simulink library "Lib_Dyn_StateSpace_TMATS"  (R2017a)
settings: Solver=ode45  StartTime=0.0  StopTime=10.0  RelTol=1e-3  EnableMultiTasking=on
Description:
  | Thomas Modules
settings Model: Creator=jwchapm2  LastModifiedBy=glthoma1
settings DataIOCC: LimitDataPoints=on  SaveFormat=Array
settings OptimizationCC: ExpressionDepthLimit=2147483647  LifeSpan=inf
settings DebuggingCC: UnderspecifiedInitializationDetection=Classic  MergeDetectMultiDrivingBlocksExec=none  SolverPrmCheckMsg=warning  StateNameClashWarn=warning  SFUnexpectedBacktrackingDiag=warning  SFNoUnconditionalDefaultTransitionDiag=warning  SFExecutionAtInitializationDiag=none
settings HardwareCC: ProdBitPerPointer=32  ProdBitPerSizeT=32  ProdBitPerPtrDiffT=32  ProdLargestAtomicFloat=None  ProdIntDivRoundTo=Undefined  ProdEndianess=Unspecified  ProdWordSize=32  ProdHWDeviceType=32-bit Generic
settings ModelReferenceCC: PropagateSignalLabelsOutOfModel=off
settings GRTTargetCC: TargetLangStandard=C89/C90 (ANSI)  GeneratePreprocessorConditionals=Disable all
settings ConfigComp: CovMetricSettings=dw  CovHtmlReporting=on  CovSaveCumulativeToWorkspaceVar=on  CovSaveSingleToWorkspaceVar=on  CovExternalEMLEnable=off

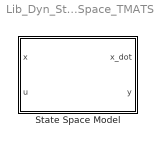
== system Lib_Dyn_StateSpace_TMATS ==
  State Space Model : Subsystem  mask(State Space Model){A_M=-1, B_M=1, C_M=1, D_M=0}
      mask prompts: A_M "A_M - "A" Matrix"; B_M "B_M - "B" Matrix"; C_M "C_M - "C" Matrix"; D_M "D_M - "D" Matrix"
      mask help:
      | This block represents a state space model that can be placed within an interative subsytem (i.e. the Newton-Raphson solver).
      | The states, x, and inputs, u must be fed into the block. The outputs, y, and state derivatives, x_dot are computed
      | via the standard state space equations. Note that the integrator that computes the states by integrating
      | the state derivatives should be placed outside of the iterative subsystem so that multiple integration steps do not
      | occur per each timestep.
      |
      | Initial conditions must be specified in the integrator blocks, and ABCD matrices specified as block mask parameters.
      mask Display:
      | fprintf('x_dot = Ax+Bu\ny = Cx+Du')
      | port_label('input',1,'x')
      | port_label('input',2,'u')
      | port_label('output',1,'x_dot')
      | port_label('output',2,'y')

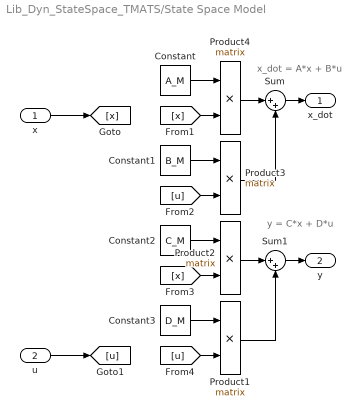
== system Lib_Dyn_StateSpace_TMATS/State Space Model ==
  note: y = C*x + D*u
  note: x_dot = A*x + B*u
  x : Inport
  u : Inport  Port=2
  Constant : Constant  Value=A_M  VectorParams1D=off
  Constant1 : Constant  Value=B_M  VectorParams1D=off
  Constant2 : Constant  Value=C_M  VectorParams1D=off
  Constant3 : Constant  Value=D_M  VectorParams1D=off
  Product{1..4} (4 alike) : Product  Multiplication=Matrix(*)
  Sum : Sum  Inputs=|++
  Sum1 : Sum  Inputs=|++
  x_dot : Outport
  y : Outport  Port=2
  wires:
  Sum/1 -> x_dot/1
  x/1 -> [x]
  Sum1/1 -> y/1
  u/1 -> [u]
  Constant/1 -> Product4/1
  [x] -> Product4/2
  [u] -> Product3/2
  Constant1/1 -> Product3/1
  Product4/1 -> Sum/1
  Product3/1 -> Sum/2
  Product2/1 -> Sum1/1
  Constant3/1 -> Product1/1
  [x] -> Product2/2
  Product1/1 -> Sum1/2
  [u] -> Product1/2
  Constant2/1 -> Product2/1
